simulink model "Timer"  (Simulink 10.0)
settings: Solver=ode1  StartTime=0.0  StopTime=inf  FixedStep=0.01  MaxStep=0.02  RelTol=1e-3  AbsTol=1e-6
libraries: simulink x2
settings Model: Creator=Admin  LastModifiedBy=bhisma  SimulationMode=external
settings ConfigSet: Description=rtmc9s12target_R2009b
settings SolverCC: AutoScaleAbsTol=off
settings DataIOCC: SignalLoggingSaveFormat=ModelDataLogs  SaveOutput=off  SaveTime=off  SignalLoggingName=sigsOut
settings OptimizationCC: BlockReduction=off  BooleanDataType=off  ExpressionDepthLimit=2147483647  InitFltsAndDblsToZero=on  LifeSpan=1  EfficientTunableParamExpr=on
settings DebuggingCC: SaveWithParameterizedLinksMsg=none  SignalResolutionControl=TryResolveAllWithWarning  MultiTaskDSMMsg=warning  MultiTaskCondExecSysMsg=none  FcnCallInpInsideContextMsg=warning  StateNameClashWarn=warning
settings HardwareCC: ProdBitPerInt=16  ProdBitPerPointer=16  ProdBitPerSizeT=16  ProdBitPerPtrDiffT=16  ProdEndianess=BigEndian  ProdWordSize=16  ProdHWDeviceType=Motorola HC12
settings SFSimCC: MATLABDynamicMemAlloc=off
settings RTWCC: SystemTargetFile=mc9s12.tlc  GenerateMakefile=off  TemplateMakefile=mc9s12.tmf
settings CodeAppCC: IgnoreCustomStorageClasses=off  CustomSymbolStrType=$N$R$M  InternalIdentifier=Classic
settings STFCustomTargetCC: TargetFcnLib=ansi_tfl_tmw.mat  ModelReferenceCompliant=off  IncludeMdlTerminateFcn=off  ERTCustomFileBanners=on  SupportNonInlinedSFcns=off  RemoveResetFunc=on  MATLABClassNameForMDSCustomization=Simulink.SoftwareTarget.ERTCustomization  CPPClassGenCompliant=on  SystemTargetFile=mc9s12.tlc
settings ERTTargetCC: TargetFcnLib=ansi_tfl_tmw.mat  MultiwordLength=2048  ModelReferenceCompliant=off  ParMdlRefBuildCompliant=off  CompOptLevelCompliant=off  ConcurrentExecutionCompliant=off  IncludeMdlTerminateFcn=off  CombineOutputUpdateFcns=off  SupportContinuousTime=on  ModelStepFunctionPrototypeControlCompliant=off  GRTInterface=on  UseToolchainInfoCompliant=off  ExtMode=on  ExtModeMexFile=ext_serial_mc9s12_comm  ExtModeMexArgs=1,2,115200  ERTCustomFileTemplate=mc9s12_file_process.tlc  ConvertIfToSwitch=off  SuppressUnreachableDefaultCases=off
settings CustomProperty: DataType=RTWOptions_EnumType_C__Users_fw__SVN_rtmc9s12-target_trunk_rtmc9s12_CW_R2009b_bin_mc9s12_1mc9s12_TargetBoard  Value=Dragon12Plus
settings EnumStrPairs: String=Dragon12
settings ConfigComp: CovExternalEMLEnable=off

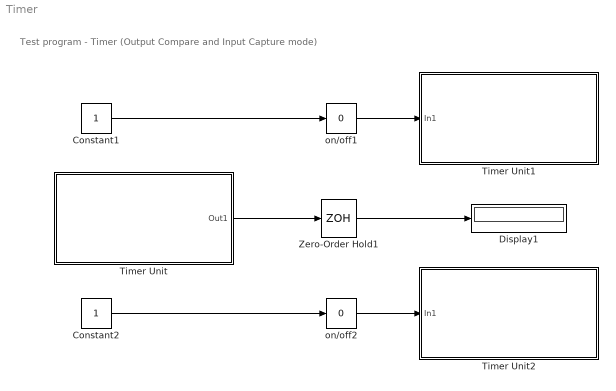
== system Timer ==
  note: Test program - Timer (Output Compare and Input Capture mode)
  Constant1 : Constant
  Constant2 : Constant
  Display1 : Display
  Timer Unit : Subsystem  Tag=mcTarget_timer  mask{timerChannel=Channel 3, timerMode=Input Capture, timerPeriod=0.3, sampletime=0.1}
      mask prompts: timerChannel "Timer channel"; timerMode "Timer mode"; timerPeriod "Timer base period (seconds)"; sampletime "Sample time"
      mask init:
      | if(timerMode == 1)
      | 	% OC
      | 	timerPeriodTypestr = 'Period:';
      | else
      | 	% IC
      | 	timerPeriodTypestr = 'Measurement intvl:';
      | end
      | 
      | [timerChannelstr, timerModestr, timerPeriodstr, ECTResolutionstr] = mbc_timer(timerChannel, timerMode, timerPeriod, sampletime);
      | 
      | % future extension: allow for output port / pin selection
      | % this hasn't been implemented yet, as it would require the 
      | % interrupt service handlers to be configured by TLC
      | % fw-09-06
      | %
      | % the following code assumes that timerOCport and timerOCpin have been defined similarly to what's done in mbc_ditaloutput.m
      | % the function also returns two more parameters (timerPORTstr, timerPINstr)
      | % these can be used in the Icon page. Replace that line by the following:
      | % fprintf('Channel: %s\nMode: %s\n%sPeriod: %s\nResolution: %s', timerChannelstr, timerModestr, timerOptPORTstr, timerPeriodstr, ECTResolutionstr)
      | % 
      | % [timerChannelstr, timerModestr, timerPORTstr, timerPINstr, timerPeriodstr, ECTResolutionstr] = mbc_timer(timerChannel, timerMode, timerOCport, timerOCpin, timerPeriod, sampletime);
      | % 
      | % if(timerMode == 1)
      | % 	% OC -> display port / pin
      | % 	timerOptPORTstr = ['Toggle: ' timerPORTstr ', Pin(s): ' timerPINstr '\n'];
      | % else
      | % 	% IC -> don't display port / pin
      | % 	timerOptPORTstr = '';
      | % end
      mask Help: web('timer_sfcn_9S12.html');
      mask TypeOptions timerChannel: Channel 0 | Channel 1 | Channel 2 | Channel 3 | Channel 4 | Channel 5 | Channel 6
      mask TypeOptions timerMode: Output Compare | Input Capture
      mask Display: fprintf('Channel: %s\nMode: %s\nPeriod: %s\nResolution: %s', timerChannelstr, timerModestr, timerPeriodstr, ECTResolutionstr)
  Timer Unit1 : Subsystem  Tag=mcTarget_timer  mask{timerChannel=Channel 1, timerMode=Output Compare, timerPeriod=0.3, sampletime=0.1}
      mask prompts: timerChannel "Timer channel"; timerMode "Timer mode"; timerPeriod "Timer base period (seconds)"; sampletime "Sample time"
      mask init: same as Timer/Timer Unit
      mask Help: web('timer_sfcn_9S12.html');
      mask TypeOptions timerChannel: Channel 0 | Channel 1 | Channel 2 | Channel 3 | Channel 4 | Channel 5 | Channel 6
      mask TypeOptions timerMode: Output Compare | Input Capture
      mask Display: fprintf('Channel: %s\nMode: %s\nPeriod: %s\nResolution: %s', timerChannelstr, timerModestr, timerPeriodstr, ECTResolutionstr)
  Timer Unit2 : Subsystem  Tag=mcTarget_timer  mask{timerChannel=Channel 2, timerMode=Output Compare, timerPeriod=0.0001, sampletime=0.1}
      mask prompts: timerChannel "Timer channel"; timerMode "Timer mode"; timerPeriod "Timer base period (seconds)"; sampletime "Sample time"
      mask init: same as Timer/Timer Unit
      mask Help: web('timer_sfcn_9S12.html');
      mask TypeOptions timerChannel: Channel 0 | Channel 1 | Channel 2 | Channel 3 | Channel 4 | Channel 5 | Channel 6
      mask TypeOptions timerMode: Output Compare | Input Capture
      mask Display: fprintf('Channel: %s\nMode: %s\nPeriod: %s\nResolution: %s', timerChannelstr, timerModestr, timerPeriodstr, ECTResolutionstr)
  Zero-Order Hold1 : ZeroOrderHold  SampleTime=0.1
  on/off1 : simulink/Math Operations/Slider Gain  SystemSampleTime=-1  low=0  gain=0  high=1
  on/off2 : simulink/Math Operations/Slider Gain  SystemSampleTime=-1  low=0  gain=0  high=1
  wires:
  Zero-Order Hold1/1 -> Display1/1
  Timer Unit/1(Out1) -> Zero-Order Hold1/1
  Constant1/1 -> on/off1/1
  on/off1/1 -> Timer Unit1/1(In1)
  Constant2/1 -> on/off2/1
  on/off2/1 -> Timer Unit2/1(In1)

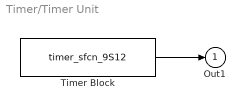
== system Timer/Timer Unit ==
  Timer Block : S-Function  Tag=mcTarget_timer  FunctionName=timer_sfcn_9S12  Parameters=sampletime, timerMode  SFunctionDeploymentMode=off  EnableBusSupport=off
  Out1 : Outport
  wires:
  Timer Block/1 -> Out1/1

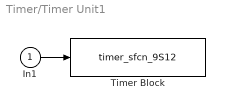
== system Timer/Timer Unit1 ==
  In1 : Inport
  Timer Block : S-Function  Tag=mcTarget_timer  FunctionName=timer_sfcn_9S12  Parameters=sampletime, timerMode  SFunctionDeploymentMode=off  EnableBusSupport=off
  wires:
  In1/1 -> Timer Block/1

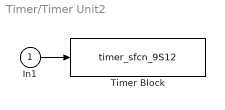
== system Timer/Timer Unit2 ==
  In1 : Inport
  Timer Block : S-Function  Tag=mcTarget_timer  FunctionName=timer_sfcn_9S12  Parameters=sampletime, timerMode  SFunctionDeploymentMode=off  EnableBusSupport=off
  wires:
  In1/1 -> Timer Block/1
